simulink subsystem "massBalance"  (R2024a)
settings: Solver=VariableStepAuto  StartTime=0.0  StopTime=7*24*3600 + 1  RelTol=1e-3
undefined symbols (not defined in the file): bath_area, concentrate_density, matte_density, offgas_fraction, slag_density
settings Model: DataDictionary=constants.sldd  EnableAccessToBaseWorkspace=off  DefaultTestHarness=massBalance_HarnessFromWorkspace  Creator=eunice.duplessis  LastModifiedBy=jason.miskin

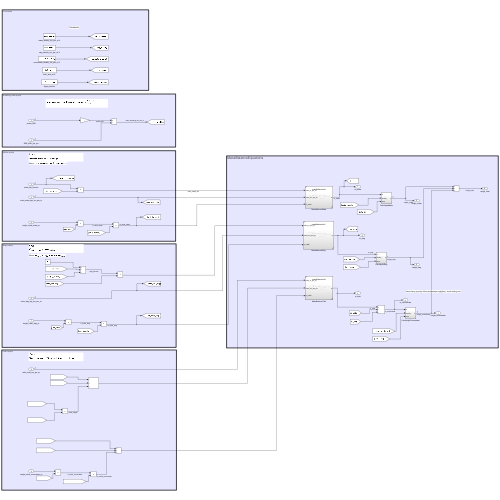
[thumbnail: Simulink's stored preview of the top-level diagram]
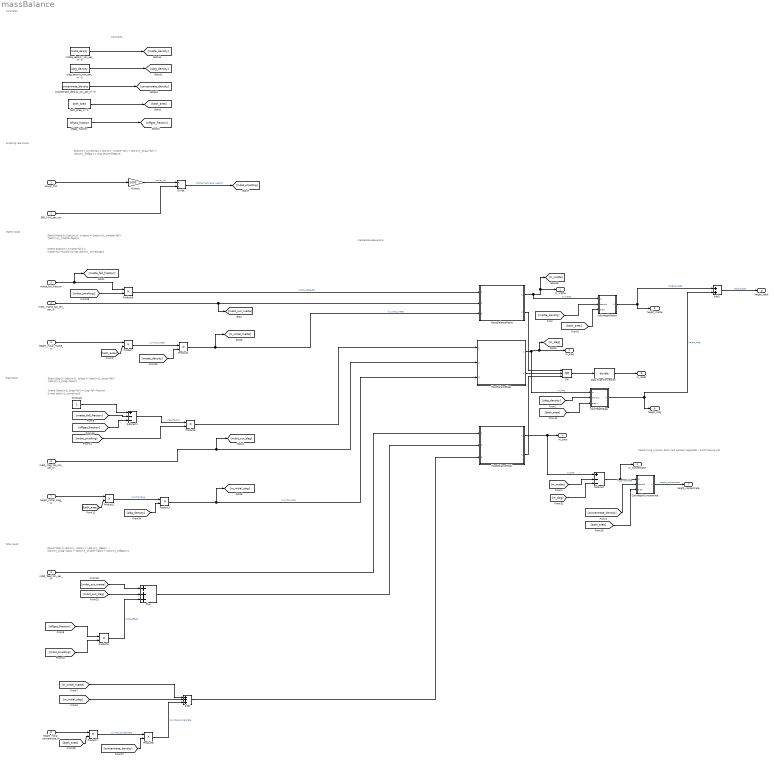
== system massBalance ==
  note: Total inputs
  note: Slag inputs
  note: Matte inputs
  note: Smelting rate inputs
  note: Constants
  note: MassBalanceEquations
  note: Where: $\dot{m}_{matte~fall} = matte~fall~fraction \times \dot{m}_{smelting}$
  note: Constants
  note: $\text{Slag:}\\ {\dot{m}}_{slag} = {\dot{m}}_{slag~fall} - {\dot{m}}_{slag~taps}$
  note: Where: $\dot{m}_{slag~fall} = slag~fall~fraction \times \dot{m}_{smelting}$
  note: $\text{Matte:}\\ {\dot{m}}_{matte} = {\dot{m}}_{matte~fall} - {\dot{m}}_{matte~taps}$
  note: $\dot{m}_{smelting} = \dot{m}_{matte~fall} + \dot{m}_{slag~fall} + \dot{m}_{offgas} = \frac{Power}{SEC}$
  note: $\text{Total:}\\ \dot{m}_{total} = (\dot{m}_{feed}) - ( \dot{m}_{slag~taps} + \dot{m}_{matte~taps} + \dot{m}_{offgas})$
  note: freeze lining: typically 30cm (but perhaps negligible) - worth looking into
  power_MW : Inport
  SER_kWh_per_ton : Inport  Port=2
  matte_fall_fraction : Inport  Port=3
  mdot_matte_tap_ton_per_hr : Inport  Port=4
  height_initial_matte_m : Inport  Port=5
  mdot_slag_tap_ton_per_hr : Inport  Port=6
  height_initial_slag_m : Inport  Port=7
  mdot_feed_ton_per_hr : Inport  Port=8
  height_initial_concentrate_m : Inport  Port=9
  Add1 : Sum
  Add2 : Sum  Inputs=+++
  CalcHeightConcentrate : Subsystem
  CalcHeightMatte : Subsystem
  CalcHeightSlag : Subsystem
  Constant : Constant
  Data Type Conversion : DataTypeConversion  OutDataTypeStr=double  SaturateOnIntegerOverflow=off  RndMeth=Floor
  Divide : Product  Inputs=*/
  MassBalanceMatte : Subsystem  ReferencedSubsystem=massBalanceUnit
  MassBalanceSlag : Subsystem  ReferencedSubsystem=massBalanceUnit
  MassBalanceTotal : Subsystem  ReferencedSubsystem=massBalanceUnit
  Multiply : Gain  Gain=1000
  OR : Logic  Operator=OR  Inputs=3  IconShape=distinctive  AllPortsSameDT=off  OutDataTypeStr=boolean
  Plus : Sum  Inputs=+++
  Product{,1..3,5..9} (9 alike) : Product
  Subtract : Sum  Inputs=+--
  Subtract1 : Sum  Inputs=+--
  bath_area_m^2 : Constant  Value=bath_area
  concentrate_density_ton_per_m^3 : Constant  Value=concentrate_density
  matte_density_ton_per_m^3 : Constant  Value=matte_density
  offgas_fraction : Constant  Value=offgas_fraction
  slag_density_ton_per_m^3 : Constant  Value=slag_density
  m_matte : Outport
  m_slag : Outport  Port=2
  m_concentrate : Outport  Port=3
  m_total : Outport  Port=4
  height_matte : Outport  Port=5
  height_slag : Outport  Port=6
  height_concentrate : Outport  Port=7
  height_total : Outport  Port=8
  is_reset : Outport  Port=9
  wires:
  [slag_density] -> CalcHeightSlag/2(density)
  [bath_area] -> CalcHeightSlag/3(area)
  MassBalanceSlag/1 -> [m_slag], m_slag/1, CalcHeightSlag/1(m)  "m_slag"
  CalcHeightSlag/1(h) -> Add1/2, height_slag/1  "height_slag"
  Product6/1 -> MassBalanceSlag/1
  mdot_slag_tap_ton_per_hr/1 -> [mdot_out_slag], MassBalanceSlag/2
  MassBalanceMatte/1 -> m_matte/1, [m_matte], CalcHeightMatte/1(m)  "m_matte"
  CalcHeightMatte/1(h) -> Add1/1, height_matte/1  "height_matte"
  mdot_matte_tap_ton_per_hr/1 -> [mdot_out_matte], MassBalanceMatte/2
  [bath_area] -> CalcHeightMatte/3(area)
  [matte_density] -> CalcHeightMatte/2(density)
  Add1/1 -> height_total/1  "height_total"
  power_MW/1 -> Multiply/1
  bath_area_m^2/1 -> [bath_area]
  [mdot_out_slag] -> Plus/2
  Multiply/1 -> Divide/1  "power_kW"
  Product5/1 -> Plus/3  "mdot_offgas"
  [matte_density] -> Product1/2
  concentrate_density_ton_per_m^3/1 -> [concentrate_density]
  [bath_area] -> Product7/2
  Product7/1 -> Product8/1  "V_initial_concentrate"
  Divide/1 -> [mdot_smelting]  "mdot_smelting_ton_per_hr"
  [bath_area] -> Product/2
  [offgas_fraction] -> Subtract1/3
  Product2/1 -> Product3/1  "V_initial_slag"
  Subtract1/1 -> Product6/1  "slag_fraction"
  [concentrate_density] -> Product8/2
  slag_density_ton_per_m^3/1 -> [slag_density]
  matte_density_ton_per_m^3/1 -> [matte_density]
  [mdot_smelting] -> Product5/2
  Product1/1 -> [m_initial_matte], MassBalanceMatte/3  "m_initial_matte"
  Constant/1 -> Subtract1/1
  height_initial_concentrate_m/1 -> Product7/1
  [slag_density] -> Product3/2
  height_initial_slag_m/1 -> Product2/1
  [bath_area] -> Product2/2
  height_initial_matte_m/1 -> Product/1
  Product8/1 -> Add2/3  "m_initial_concentrate"
  offgas_fraction/1 -> [offgas_fraction]
  Product/1 -> Product1/1  "V_initial_matte"
  [m_initial_matte] -> Add2/1
  [m_initial_slag] -> Add2/2
  Product3/1 -> [m_initial_slag], MassBalanceSlag/3  "m_initial_slag"
  [offgas_fraction] -> Product5/1
  [matte_fall_fraction] -> Subtract1/2
  [mdot_out_matte] -> Plus/1
  SER_kWh_per_ton/1 -> Divide/2
  [mdot_smelting] -> Product6/2
  Plus/1 -> MassBalanceTotal/2
  CalcHeightConcentrate/1(h) -> height_concentrate/1  "height_concentrate"
  Add2/1 -> MassBalanceTotal/3
  [bath_area] -> CalcHeightConcentrate/3(area)
  mdot_feed_ton_per_hr/1 -> MassBalanceTotal/1
  [concentrate_density] -> CalcHeightConcentrate/2(density)
  MassBalanceTotal/1 -> m_total/1, Subtract/1  "m_total"
  Subtract/1 -> CalcHeightConcentrate/1(m), m_concentrate/1  "m_concentrate"
  [m_matte] -> Subtract/2
  [m_slag] -> Subtract/3
  matte_fall_fraction/1 -> [matte_fall_fraction], Product9/1
  [mdot_smelting] -> Product9/2
  Product9/1 -> MassBalanceMatte/1  "mdot_matte_fall"
  OR/1 -> Data Type Conversion/1
  MassBalanceMatte/2 -> OR/1
  MassBalanceSlag/2 -> OR/2
  MassBalanceTotal/2 -> OR/3
  Data Type Conversion/1 -> is_reset/1

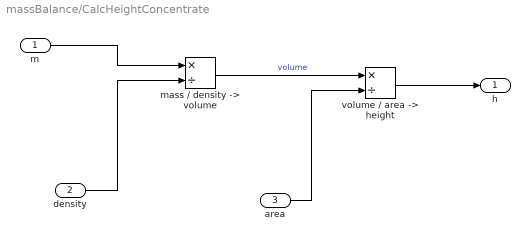
== system massBalance/CalcHeightConcentrate ==
  m : Inport
  density : Inport  Port=2
  area : Inport  Port=3
  "mass / density -> volume" : Product  Inputs=*/
  "volume / area -> height" : Product  Inputs=*/
  h : Outport
  wires:
  "mass / density -> volume"/1 -> "volume / area -> height"/1  "volume"
  density/1 -> "mass / density -> volume"/2
  "volume / area -> height"/1 -> h/1
  m/1 -> "mass / density -> volume"/1
  area/1 -> "volume / area -> height"/2

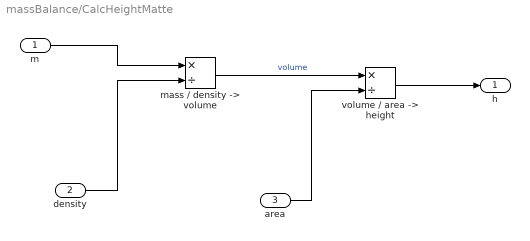
== system massBalance/CalcHeightMatte ==
  m : Inport
  density : Inport  Port=2
  area : Inport  Port=3
  "mass / density -> volume" : Product  Inputs=*/
  "volume / area -> height" : Product  Inputs=*/
  h : Outport
  wires:
  area/1 -> "volume / area -> height"/2
  m/1 -> "mass / density -> volume"/1
  "volume / area -> height"/1 -> h/1
  density/1 -> "mass / density -> volume"/2
  "mass / density -> volume"/1 -> "volume / area -> height"/1  "volume"

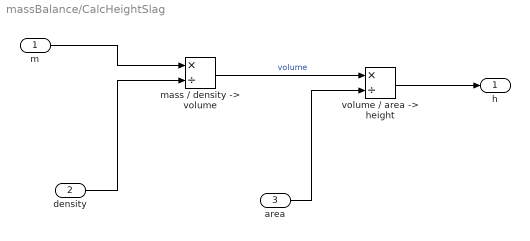
== system massBalance/CalcHeightSlag ==
  m : Inport
  density : Inport  Port=2
  area : Inport  Port=3
  "mass / density -> volume" : Product  Inputs=*/
  "volume / area -> height" : Product  Inputs=*/
  h : Outport
  wires:
  "mass / density -> volume"/1 -> "volume / area -> height"/1  "volume"
  density/1 -> "mass / density -> volume"/2
  "volume / area -> height"/1 -> h/1
  m/1 -> "mass / density -> volume"/1
  area/1 -> "volume / area -> height"/2
